simulink model "power_wind_dfig"  (R2016a)
settings: Solver=ode23tb  StartTime=0.0  StopTime=100  FixedStep=1/60  MaxStep=1/60  RelTol=1e-4  AbsTol=1e-3
InitFcn:
  | xInitial = init_power_wind_dfig;
undefined symbols (not defined in the file): b0, D1, D11, Delta, F, find_system, Fnom, gcbh, H, ILd_init, ILq_init, Imax_grid_conv, Init, j, Kd, Ki_dc_reg, Ki_grid_side_cur_reg, Ki_power_reg, Ki_Q, Ki_rotor_side_cur_reg, Ki_volt_reg, Kp, Kp_dc_reg, Kp_grid_side_cur_reg, Kp_power_reg, Kp_Q, Kp_rotor_side_cur_reg, Kp_volt_reg, L_RL, Llr, Lls, p, Pnom, power_A, power_B, power_D, R_RL, Rr, Rs, speed_A, speed_B, speed_C, speed_D, sps_rtmsupport, Vcontrol, Vnom, Wind_On, wo
libraries: powerlib_meascontrol x29, powerlib x27, simulink_extras x5, re_lib x2
(part 2 of 5)

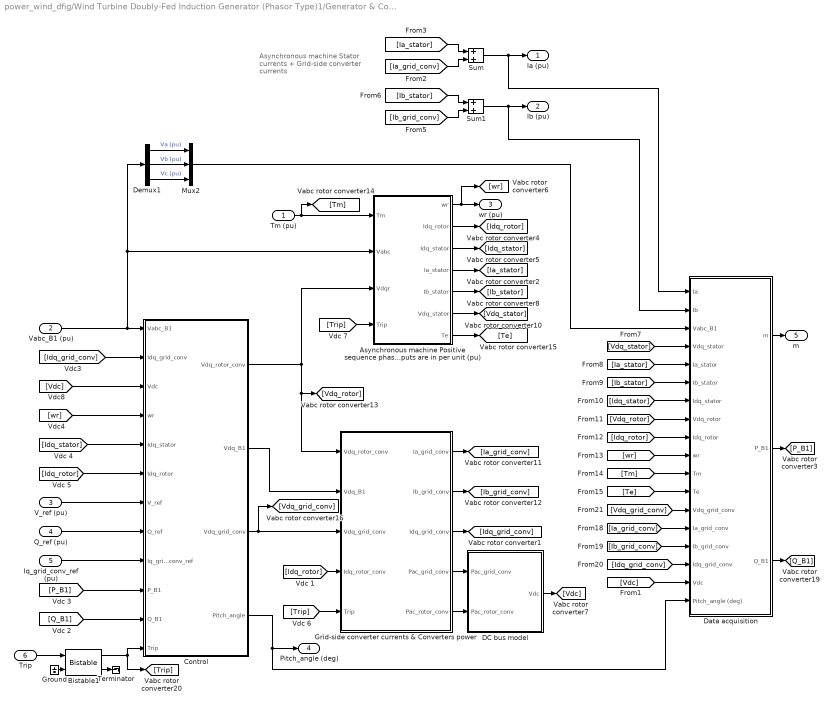
== system power_wind_dfig/Wind Turbine Doubly-Fed Induction Generator (Phasor Type)1/Generator & Converters ==
  note: Asynchronous machine
      | Stator currents
      | +
      | Grid-side converter
      | currents
  Tm (pu) : Inport
  Vabc_B1 (pu) : Inport  Port=2
  V_ref (pu) : Inport  Port=3
  Q_ref (pu) : Inport  Port=4
  Iq_grid_conv_ref (pu) : Inport  Port=5
  Trip : Inport  Port=6
  Asynchronous machine Positive sequence phasor model Inputs and outputs are in per unit (pu) : Subsystem  mask(Asynchronous Machine Model){nom=[ Pnom Vnom Fnom ], sta=[ Rs Lls], rot=[ Rr Llr], Lm=Lm, mec=[H F p], ini=init}
      mask prompts: nom "Nom. power,L-L volt. and freq. [ Pn(VA),Vn(Vrms),fn(Hz) ]:"; sta "Stator [ Rs,Lls (pu) ]:"; rot "Rotor [ Rr',Llr' (pu) ]:"; Lm "Magnetizing inductance Lm (pu):"; mec "Inertia constant,friction factor and pairs of poles [ H(s)  F(pu)  p() ]:"; ini "Initial conditions [s()  th(deg)  Is(pu)  ph_Is(deg)  Ir(pu)  ph_Ir(deg)]:"
      mask help: Implements a three-phase asynchronous machine (wound rotor) modelled in the dq stator reference frame. Stator and rotor windings are connected in wye to an internal neutral point.
      mask init:
      | %Initializes the Asynchronous Machine block before simulation.
      | 
      | % Base angular frequency
      | web=nom(3)*2*pi;
      | 
      | Rs=sta(1); Lls=sta(2);		% stator resistance and leakage inductance
      | Rr=rot(1); Llr=rot(2);		% rotor resistance and leakage inductance
      | Lm=Lm(1);			        % mutual inductance
      | H=mec(1); F=mec(2); p=mec(3);	% inertia, friction and pole pairs
      | s=ini(1);			% initial slip
      | wmo=1-s;			% initial speed
      | tho=ini(2)*pi/180;		% initial rotor angle
      | 
      | iso_mag=ini(3); iso_ph=ini(4)*pi/180; % init. stator current, phase A
      | iro_mag=ini(5); iro_ph=ini(6)*pi/180; % init. rotor current, phase A
      | 
      | % conversion of initial stator and rotor currents from polar to rectangular
      | % coordinates
      | [isdo,isqo]=pol2cart(iso_ph,iso_mag);
      | [irdo,irqo]=pol2cart(iro_ph,iro_mag);
      | 
      | % Initial fluxes (pu): inductances in pu, currents in pu
      | phisqo=((Lls+Lm)*isqo+Lm*irqo);
      | phisdo=((Lls+Lm)*isdo+Lm*irdo);
      | phirqo=((Llr+Lm)*irqo+Lm*isqo);
      | phirdo=((Llr+Lm)*irdo+Lm*isdo);
      | 
      | % Other inductances -------------------------------------------------------
      | 
      | Laq=1/(1/Lm+1/Lls+1/Llr);
      | Lad=Laq;
      mask Help: First 3 inputs: Stator terminals = phases a, b and c; 4th input: Simulink signal = Mechanical torque applied to the shaft (pu, >0 for motor mode, <0 for generator mode); First 3 outputs: Rotor terminals = phases a, b and c; 4th output: Simulink measurement output = vector (20x1) containing the following (all currents flowing into the machine): [1-3] : Rotor line currents ira, irb and irc; [4-5] : Rotor currents iqr and idr; [6-7] : Rotor fluxes phiqr and  phidr; [8-9] : Rotor voltages vqr and vdr; [10-12] : Stator line currents isa, isb, isc; [13-14] : Stator currents iqs and ids; [15-16] : Stator fluxes phiqs and  phids; [17-18] : Stator voltages vqs and vds; [19] : Rotor speed wm; [20 ]: Electromagnetic torque Te. Units of output measurement depend on checkbox in block's dialog box.
  Bistable1 : powerlib_meascontrol/Logic/Bistable  Qpriority=Set  ic=0  Ts=0
  Control : Subsystem
  DC bus model : Subsystem  mask(DC bus model){Pnom=Pnom, C=capacitor, Vdc_Init=Vdc_nom}
      mask prompts: Pnom "Nominal power (W):"; C "Capacitor (F):"; Vdc_Init "Initial voltage (V):"
  Data acquisition : Subsystem
  Demux1 : Demux  Outputs=3
  Grid-side converter currents & Converters power : Subsystem
  Ground : Ground
  Mux2 : Mux  Inputs=3
  Sum : Sum  SaturateOnIntegerOverflow=on
  Sum1 : Sum  SaturateOnIntegerOverflow=on
  Terminator : Terminator
  Ia (pu) : Outport
  Ib (pu) : Outport  Port=2
  wr (pu) : Outport  Port=3
  Pitch_angle (deg) : Outport  Port=4
  m : Outport  Port=5
  wires:
  Control/4(Pitch_angle) -> Pitch_angle (deg)/1, Data acquisition/18(Pitch_angle (deg))
  Bistable1/1 -> Control/12(Trip), [Trip]
  Ground/1 -> Bistable1/2
  Bistable1/2 -> Terminator/1
  Trip/1 -> Bistable1/1
  [Trip] -> Asynchronous machine Positive sequence phasor model Inputs and outputs are in per unit (pu)/4(Trip)
  [Trip] -> Grid-side converter currents & Converters power/5(Trip)
  V_ref (pu)/1 -> Control/7(V_ref)
  [Q_B1] -> Control/11(Q_B1)
  [P_B1] -> Control/10(P_B1)
  Data acquisition/2(P_B1) -> [P_B1]
  Iq_grid_conv_ref (pu)/1 -> Control/9(Iq_grid_conv_ref)
  Q_ref (pu)/1 -> Control/8(Q_ref)
  Data acquisition/3(Q_B1) -> [Q_B1]
  Demux1/3 -> Mux2/3  "Vc (pu)"
  Mux2/1 -> Data acquisition/3(Vabc_B1)
  Demux1/2 -> Mux2/2  "Vb (pu)"
  Demux1/1 -> Mux2/1  "Va (pu)"
  [Vdc] -> Data acquisition/17(Vdc)
  Data acquisition/1(m) -> m/1
  [Vdq_stator] -> Data acquisition/4(Vdq_stator)
  [Ia_stator] -> Data acquisition/5(Ia_stator)
  [Ib_stator] -> Data acquisition/6(Ib_stator)
  [Idq_stator] -> Data acquisition/7(Idq_stator)
  [Vdq_rotor] -> Data acquisition/8(Vdq_rotor)
  [Idq_rotor] -> Data acquisition/9(Idq_rotor)
  [wr] -> Data acquisition/10(wr)
  [Tm] -> Data acquisition/11(Tm)
  [Te] -> Data acquisition/12(Te)
  [Vdq_grid_conv] -> Data acquisition/13(Vdq_grid_conv)
  [Ia_grid_conv] -> Data acquisition/14(Ia_grid_conv)
  [Ib_grid_conv] -> Data acquisition/15(Ib_grid_conv)
  [Idq_grid_conv] -> Data acquisition/16(Idq_grid_conv)
  Asynchronous machine Positive sequence phasor model Inputs and outputs are in per unit (pu)/7(Te) -> [Te]
  [Ib_stator] -> Sum1/1
  [Ib_grid_conv] -> Sum1/2
  [Ia_stator] -> Sum/1
  [Ia_grid_conv] -> Sum/2
  Grid-side converter currents & Converters power/2(Ib_grid_conv) -> [Ib_grid_conv]
  Grid-side converter currents & Converters power/1(Ia_grid_conv) -> [Ia_grid_conv]
  Asynchronous machine Positive sequence phasor model Inputs and outputs are in per unit (pu)/6(Vdq_stator) -> [Vdq_stator]
  Asynchronous machine Positive sequence phasor model Inputs and outputs are in per unit (pu)/1(wr) -> [wr], wr (pu)/1
  Sum1/1 -> Data acquisition/2(Ib), Ib (pu)/1
  Sum/1 -> Data acquisition/1(Ia), Ia (pu)/1
  Vabc_B1 (pu)/1 -> Demux1/1, Asynchronous machine Positive sequence phasor model Inputs and outputs are in per unit (pu)/2(Vabc), Control/1(Vabc_B1)
  Grid-side converter currents & Converters power/5(Pac_rotor_conv) -> DC bus model/2(Pac_rotor_conv)
  Grid-side converter currents & Converters power/4(Pac_grid_conv) -> DC bus model/1(Pac_grid_conv)
  [Idq_rotor] -> Grid-side converter currents & Converters power/4(Idq_rotor_conv)
  Asynchronous machine Positive sequence phasor model Inputs and outputs are in per unit (pu)/4(Ia_stator) -> [Ia_stator]
  Asynchronous machine Positive sequence phasor model Inputs and outputs are in per unit (pu)/5(Ib_stator) -> [Ib_stator]
  Tm (pu)/1 -> [Tm], Asynchronous machine Positive sequence phasor model Inputs and outputs are in per unit (pu)/1(Tm)
  Asynchronous machine Positive sequence phasor model Inputs and outputs are in per unit (pu)/2(Idq_rotor) -> [Idq_rotor]
  Asynchronous machine Positive sequence phasor model Inputs and outputs are in per unit (pu)/3(Idq_stator) -> [Idq_stator]
  [Idq_grid_conv] -> Control/2(Idq_grid_conv)
  Grid-side converter currents & Converters power/3(Idq_grid_conv) -> [Idq_grid_conv]
  Control/2(Vdq_B1) -> Grid-side converter currents & Converters power/2(Vdq_B1)
  Control/1(Vdq_rotor_conv) -> [Vdq_rotor], Grid-side converter currents & Converters power/1(Vdq_rotor_conv), Asynchronous machine Positive sequence phasor model Inputs and outputs are in per unit (pu)/3("Vdqr ")
  Control/3(Vdq_grid_conv) -> [Vdq_grid_conv], Grid-side converter currents & Converters power/3(Vdq_grid_conv)
  [wr] -> Control/4(wr)
  [Vdc] -> Control/3(Vdc)
  [Idq_stator] -> Control/5(Idq_stator)
  [Idq_rotor] -> Control/6(Idq_rotor)
  DC bus model/1(Vdc) -> [Vdc]

== system power_wind_dfig/Wind Turbine Protection/Protection System ==
  Vabc (pu) : Inport  PortDimensions=3
  Iabc (pu) : Inport  Port=2  PortDimensions=3
  Vdc (V) : Inport  Port=3  PortDimensions=1
  Reset : Inport  Port=4  PortDimensions=1
  Speed (pu) : Inport  Port=5  PortDimensions=1
  AC Current Protection : Subsystem
  AC Voltage Protection : Subsystem
  Bistable1 : powerlib_meascontrol/Logic/Bistable  Qpriority=Set  ic=0  Ts=0
  Clock : Clock
  Constant : Constant  Value=Delay_Protection
  DC Voltage Protection : Subsystem
  Decoding : Subsystem
  Encoding : Subsystem
  Logical Operator : Logic  Operator=OR  Inputs=10  AllPortsSameDT=off
  Logical Operator1 : Logic  AllPortsSameDT=off
  Logical Operator2 : Logic  Operator=NOT  AllPortsSameDT=off
  Logical Operator3 : Logic  AllPortsSameDT=off
  Memory : Memory  InheritSampleTime=on
  Memory1 : Memory  InheritSampleTime=on
  Monostable1 : powerlib_meascontrol/Logic/Monostable  EdgeDetect=Rising  PulseDuration=1e-9  ic=0  Ts=0
  Relational Operator10 : RelationalOperator
  Sample & Hold : Subsystem  DialogController=POWERSYS.PowerSysDialog  mask(Sample & Hold){ic=0}
      mask prompts: ic "Initial condition:"
      mask help: The output follows input 1 (In) as long as input 2 (S) is TRUE (1) . The output is held when input 2 becomes FALSE (0). The output initial value is specified by the parameter "Initial condition".
      mask init:
      | power_initmask();
      mask Help: This block is part of a subset of blocks in the Extras library that does not have documentation associated with it, other than the block mask description.
      mask Display: disp('S/H')
  Sample & Hold1 : Subsystem  DialogController=POWERSYS.PowerSysDialog  mask(Sample & Hold){ic=0}
      mask prompts: ic "Initial condition:"
      mask help: The output follows input 1 (In) as long as input 2 (S) is TRUE (1) . The output is held when input 2 becomes FALSE (0). The output initial value is specified by the parameter "Initial condition".
      mask init:
      | power_initmask();
      mask Help: This block is part of a subset of blocks in the Extras library that does not have documentation associated with it, other than the block mask description.
      mask Display: disp('S/H')
  Terminator : Terminator
  Under/Over Speed Protection : Subsystem
  Trip : Outport
  TripTime : Outport  Port=2
  TripStatus : Outport  Port=3
  wires:
  Speed (pu)/1 -> Under/Over Speed Protection/1(Speed)
  Under/Over Speed Protection/2(MaxSpeed) -> Encoding/10(In10), Logical Operator/10
  Under/Over Speed Protection/1(MinSpeed) -> Encoding/9(In9), Logical Operator/9
  Relational Operator10/1 -> Logical Operator1/2
  Logical Operator/1 -> Logical Operator1/1
  Clock/1 -> Sample & Hold1/1(In), Relational Operator10/1
  Constant/1 -> Relational Operator10/2
  Monostable1/1 -> Sample & Hold1/2(S), Sample & Hold/2(S)
  Sample & Hold1/1("   ") -> TripTime/1
  AC Voltage Protection/4(MaxV0V1) -> Encoding/7(In7), Logical Operator/7
  AC Voltage Protection/3(MaxV2V1) -> Encoding/6(In6), Logical Operator/6
  AC Voltage Protection/2(MaxV1) -> Encoding/5(In5), Logical Operator/5
  AC Voltage Protection/1(MinV1) -> Encoding/4(In4), Logical Operator/4
  AC Current Protection/3(MaxI2I1) -> Encoding/3(In3), Logical Operator/3
  AC Current Protection/2(MaxI1) -> Encoding/2(In2), Logical Operator/2
  AC Current Protection/1(MaxIinst) -> Encoding/1(In1), Logical Operator/1
  Vabc (pu)/1 -> AC Voltage Protection/1(abc)
  Iabc (pu)/1 -> AC Current Protection/1(abc)
  Decoding/1(Out) -> TripStatus/1
  Sample & Hold/1("   ") -> Decoding/1(Code)
  Bistable1/2 -> Terminator/1
  Memory/1 -> Monostable1/1, Memory1/1
  Bistable1/1 -> Memory/1
  Encoding/1(Code) -> Sample & Hold/1(In)
  Logical Operator1/1 -> Bistable1/1, Logical Operator2/1
  Logical Operator3/1 -> Bistable1/2
  Reset/1 -> Logical Operator3/2
  Logical Operator2/1 -> Logical Operator3/1
  DC Voltage Protection/1(MaxVdc) -> Encoding/8(In8), Logical Operator/8
  Vdc (V)/1 -> DC Voltage Protection/1(Vdc)
  Memory1/1 -> Trip/1

== system power_wind_dfig/Measurements/Grid Data acquisition/Mean Value1 ==
  note: Mean value
  In : Inport
  Init : Inport  Port=2
  Gain : Gain  Gain=1/Period  SaturateOnIntegerOverflow=on  OutDataTypeStr=Inherit: Same as input  ParamDataTypeStr=Inherit: Same as input
  Step : Step  Time=Period+eps  SampleTime=0
  Sum : Sum  Inputs=+-  SaturateOnIntegerOverflow=on  InputSameDT=on  OutDataTypeStr=Inherit: Same as first input
  Switch : Switch  Threshold=0.5  SaturateOnIntegerOverflow=on
  Transport Delay : TransportDelay  DelayTime=Period
  integrator : Integrator
  Mean : Outport
  wires:
  Transport Delay/1 -> Sum/2
  integrator/1 -> Transport Delay/1, Sum/1
  In/1 -> integrator/1
  Sum/1 -> Gain/1
  Gain/1 -> Switch/1
  Switch/1 -> Mean/1
  Step/1 -> Switch/2
  Init/1 -> Switch/3

== system power_wind_dfig/Measurements/Grid Data acquisition/Mean Value2 ==
  note: Mean value
  In : Inport
  Init : Inport  Port=2
  Gain : Gain  Gain=1/Period  SaturateOnIntegerOverflow=on  OutDataTypeStr=Inherit: Same as input  ParamDataTypeStr=Inherit: Same as input
  Step : Step  Time=Period+eps  SampleTime=0
  Sum : Sum  Inputs=+-  SaturateOnIntegerOverflow=on  InputSameDT=on  OutDataTypeStr=Inherit: Same as first input
  Switch : Switch  Threshold=0.5  SaturateOnIntegerOverflow=on
  Transport Delay : TransportDelay  DelayTime=Period
  integrator : Integrator
  Mean : Outport
  wires:
  Init/1 -> Switch/3
  Step/1 -> Switch/2
  Switch/1 -> Mean/1
  Gain/1 -> Switch/1
  Sum/1 -> Gain/1
  In/1 -> integrator/1
  integrator/1 -> Sum/1, Transport Delay/1
  Transport Delay/1 -> Sum/2

== system power_wind_dfig/Measurements/Wind turbine Data acquisition/Mean Value1 ==
  note: Mean value
  In : Inport
  Init : Inport  Port=2
  Gain : Gain  Gain=1/Period  SaturateOnIntegerOverflow=on  OutDataTypeStr=Inherit: Same as input  ParamDataTypeStr=Inherit: Same as input
  Step : Step  Time=Period+eps  SampleTime=0
  Sum : Sum  Inputs=+-  SaturateOnIntegerOverflow=on  InputSameDT=on  OutDataTypeStr=Inherit: Same as first input
  Switch : Switch  Threshold=0.5  SaturateOnIntegerOverflow=on
  Transport Delay : TransportDelay  DelayTime=Period
  integrator : Integrator
  Mean : Outport
  wires:
  Transport Delay/1 -> Sum/2
  integrator/1 -> Transport Delay/1, Sum/1
  In/1 -> integrator/1
  Sum/1 -> Gain/1
  Gain/1 -> Switch/1
  Switch/1 -> Mean/1
  Step/1 -> Switch/2
  Init/1 -> Switch/3

== system power_wind_dfig/Measurements/Wind turbine Data acquisition/Mean Value2 ==
  note: Mean value
  In : Inport
  Init : Inport  Port=2
  Gain : Gain  Gain=1/Period  SaturateOnIntegerOverflow=on  OutDataTypeStr=Inherit: Same as input  ParamDataTypeStr=Inherit: Same as input
  Step : Step  Time=Period+eps  SampleTime=0
  Sum : Sum  Inputs=+-  SaturateOnIntegerOverflow=on  InputSameDT=on  OutDataTypeStr=Inherit: Same as first input
  Switch : Switch  Threshold=0.5  SaturateOnIntegerOverflow=on
  Transport Delay : TransportDelay  DelayTime=Period
  integrator : Integrator
  Mean : Outport
  wires:
  Init/1 -> Switch/3
  Step/1 -> Switch/2
  Switch/1 -> Mean/1
  Gain/1 -> Switch/1
  Sum/1 -> Gain/1
  In/1 -> integrator/1
  integrator/1 -> Sum/1, Transport Delay/1
  Transport Delay/1 -> Sum/2

== system power_wind_dfig/Measurements/Wind turbine Data acquisition/magnitude positive seq.  ==
  In1 : Inport
  Complex to Real-Imag : ComplexToRealImag
  Fourier1 : Subsystem  mask(Fourier analyser){f1=60, n=0}
      mask prompts: f1 "Fundamental frequency f1 (Hz):"; n "Harmonic n (0=DC; 1=fundamental; 2=2nd harm;  ...) :"
      mask help: The Fourier block performs a Fourier analysis of the input signal over a running window of one cycle of the fundamental frequency. First and second outputs return respectively the magnitude and phase (degrees) of the harmonic component specified.
      mask init:
      | k=2-(n==0);
      mask Help: helpview(psbhelp)
  Fourier2 : Subsystem  mask(Fourier analyser){f1=60, n=0}
      mask prompts: f1 "Fundamental frequency f1 (Hz):"; n "Harmonic n (0=DC; 1=fundamental; 2=2nd harm;  ...) :"
      mask help: The Fourier block performs a Fourier analysis of the input signal over a running window of one cycle of the fundamental frequency. First and second outputs return respectively the magnitude and phase (degrees) of the harmonic component specified.
      mask init:
      | k=2-(n==0);
      mask Help: helpview(psbhelp)
  Math Function : Math  Operator=hypot  SaturateOnIntegerOverflow=on
  Terminator : Terminator
  Terminator1 : Terminator
  Out1 : Outport
  wires:
  In1/1 -> Complex to Real-Imag/1
  Math Function/1 -> Out1/1
  Fourier2/1(magnitude) -> Math Function/2
  Fourier1/1(magnitude) -> Math Function/1
  Fourier2/2(angle) -> Terminator1/1
  Fourier1/2(angle) -> Terminator/1
  Complex to Real-Imag/2 -> Fourier2/1(signal)
  Complex to Real-Imag/1 -> Fourier1/1(signal)

== system power_wind_dfig/Measurements/Wind turbine Data acquisition/magnitude positivie seq ==
  In1 : Inport
  Complex to Real-Imag : ComplexToRealImag
  Fourier1 : Subsystem  mask(Fourier analyser){f1=60, n=0}
      mask prompts: f1 "Fundamental frequency f1 (Hz):"; n "Harmonic n (0=DC; 1=fundamental; 2=2nd harm;  ...) :"
      mask help: The Fourier block performs a Fourier analysis of the input signal over a running window of one cycle of the fundamental frequency. First and second outputs return respectively the magnitude and phase (degrees) of the harmonic component specified.
      mask init:
      | k=2-(n==0);
      mask Help: helpview(psbhelp)
  Fourier2 : Subsystem  mask(Fourier analyser){f1=60, n=0}
      mask prompts: f1 "Fundamental frequency f1 (Hz):"; n "Harmonic n (0=DC; 1=fundamental; 2=2nd harm;  ...) :"
      mask help: The Fourier block performs a Fourier analysis of the input signal over a running window of one cycle of the fundamental frequency. First and second outputs return respectively the magnitude and phase (degrees) of the harmonic component specified.
      mask init:
      | k=2-(n==0);
      mask Help: helpview(psbhelp)
  Math Function : Math  Operator=hypot  SaturateOnIntegerOverflow=on
  Terminator : Terminator
  Terminator1 : Terminator
  Out1 : Outport
  wires:
  Complex to Real-Imag/1 -> Fourier1/1(signal)
  Complex to Real-Imag/2 -> Fourier2/1(signal)
  Fourier1/2(angle) -> Terminator/1
  Fourier2/2(angle) -> Terminator1/1
  Fourier1/1(magnitude) -> Math Function/1
  Fourier2/1(magnitude) -> Math Function/2
  Math Function/1 -> Out1/1
  In1/1 -> Complex to Real-Imag/1

== system power_wind_dfig/Plant 2 MVA/Plant & Motor Protection/AC Current Protection ==
  abc : Inport  PortDimensions=3
  Complex to Magnitude-Angle1 : ComplexToMagnitudeAngle  Output=Magnitude
  Current Measurement : Subsystem
  MinMax : MinMax  Function=max  ZeroCross=off  SaturateOnIntegerOverflow=on  InputSameDT=on
  Mux : Mux  Inputs=3
  On Delay : powerlib_meascontrol/Logic/On Delay  DelayType=On delay  delay=Delay_I1  ic=0  Ts=0
  On Delay1 : powerlib_meascontrol/Logic/On Delay  DelayType=On delay  delay=Delay_I2_I1  ic=0  Ts=0
  Relational Operator10 : RelationalOperator  Operator=>
  Relational Operator6 : RelationalOperator  Operator=>
  Relational Operator8 : RelationalOperator  Operator=>
  Selector : Selector  InputPortWidth=3  IndexOptions=Index vector (dialog)  Indices=1  OutputSizes=1
  Selector1 : Selector  InputPortWidth=3  IndexOptions=Index vector (dialog)  Indices=2  OutputSizes=1
  Selector2 : Selector  InputPortWidth=3  IndexOptions=Index vector (dialog)  Indices=3  OutputSizes=1
  V0/V1 max3 : Constant  Value=Max_I1
  V1 max : Constant  Value=Max_I2_I1
  V1 max2 : Constant  Value=Max_Iinst
  MaxIinst : Outport
  MaxI1 : Outport  Port=2
  MaxI2I1 : Outport  Port=3
  wires:
  MinMax/1 -> Relational Operator10/1
  Complex to Magnitude-Angle1/1 -> MinMax/1
  Mux/1 -> Complex to Magnitude-Angle1/1
  Selector1/1 -> Mux/2
  Selector2/1 -> Mux/3
  Selector/1 -> Mux/1
  V1 max2/1 -> Relational Operator10/2
  Relational Operator10/1 -> MaxIinst/1
  On Delay1/1 -> MaxI2I1/1
  On Delay/1 -> MaxI1/1
  Relational Operator8/1 -> On Delay1/1
  Relational Operator6/1 -> On Delay/1
  Current Measurement/2(I2/I1) -> Relational Operator8/1
  V1 max/1 -> Relational Operator8/2
  V0/V1 max3/1 -> Relational Operator6/2
  Current Measurement/1(I1) -> Relational Operator6/1
  abc/1 -> Selector2/1, Selector1/1, Selector/1, Current Measurement/1(abc)

== system power_wind_dfig/Plant 2 MVA/Plant & Motor Protection/AC Voltage Protection ==
  abc : Inport  PortDimensions=3
  On Delay : powerlib_meascontrol/Logic/On Delay  DelayType=On delay  delay=Delay_V1  ic=0  Ts=0
  On Delay1 : powerlib_meascontrol/Logic/On Delay  DelayType=On delay  delay=Delay_V2_V1  ic=0  Ts=0
  On Delay2 : powerlib_meascontrol/Logic/On Delay  DelayType=On delay  delay=Delay_V1  ic=0  Ts=0
  On Delay3 : powerlib_meascontrol/Logic/On Delay  DelayType=On delay  delay=Delay_V2_V1  ic=0  Ts=0
  Relational Operator6 : RelationalOperator  Operator=>
  Relational Operator7 : RelationalOperator  Operator=<
  Relational Operator8 : RelationalOperator  Operator=>
  Relational Operator9 : RelationalOperator  Operator=>
  V0/V1 max3 : Constant  Value=Max_V1
  V0/V1 max4 : Constant  Value=Min_V1
  V1 max : Constant  Value=Max_V2_V1
  V1 max1 : Constant  Value=Max_V0_V1
  Voltage Measurement : Subsystem
  MinV1 : Outport
  MaxV1 : Outport  Port=2
  MaxV2V1 : Outport  Port=3
  MaxV0V1 : Outport  Port=4
  wires:
  abc/1 -> Voltage Measurement/1(abc)
  Voltage Measurement/1(V1) -> Relational Operator6/1, Relational Operator7/1
  V0/V1 max3/1 -> Relational Operator6/2
  V0/V1 max4/1 -> Relational Operator7/2
  V1 max/1 -> Relational Operator8/2
  Voltage Measurement/2(V2/V1) -> Relational Operator8/1
  V1 max1/1 -> Relational Operator9/2
  Voltage Measurement/3(V0/V1) -> Relational Operator9/1
  Relational Operator6/1 -> On Delay2/1
  Relational Operator7/1 -> On Delay/1
  Relational Operator8/1 -> On Delay1/1
  Relational Operator9/1 -> On Delay3/1
  On Delay2/1 -> MaxV1/1
  On Delay/1 -> MinV1/1
  On Delay1/1 -> MaxV2V1/1
  On Delay3/1 -> MaxV0V1/1

== system power_wind_dfig/Plant 2 MVA/Plant & Motor Protection/DC Voltage Protection ==
  Vdc : Inport
  On Delay : powerlib_meascontrol/Logic/On Delay  DelayType=On delay  delay=Delay_Vdc  ic=0  Ts=0
  Relational Operator1 : RelationalOperator  Operator=>
  V1 max3 : Constant  Value=Max_Vdc
  MaxVdc : Outport
  wires:
  On Delay/1 -> MaxVdc/1
  Relational Operator1/1 -> On Delay/1
  V1 max3/1 -> Relational Operator1/2
  Vdc/1 -> Relational Operator1/1

== system power_wind_dfig/Plant 2 MVA/Plant & Motor Protection/Decoding ==
  Code : Inport
  Constant : Constant  Value=pow2(0:-1:-9)
  Constant6 : Constant  Value=2
  Math Function : Math  Operator=rem  SaturateOnIntegerOverflow=on
  Product : Product  SaturateOnIntegerOverflow=on  InputSameDT=on  OutDataTypeStr=Inherit: Same as first input
  Rounding Function : Rounding
  Out : Outport
  wires:
  Math Function/1 -> Out/1
  Rounding Function/1 -> Math Function/1
  Constant6/1 -> Math Function/2
  Product/1 -> Rounding Function/1
  Code/1 -> Product/1
  Constant/1 -> Product/2

== system power_wind_dfig/Plant 2 MVA/Plant & Motor Protection/Encoding ==
  In1 : Inport
  In2 : Inport  Port=2
  In3 : Inport  Port=3
  In4 : Inport  Port=4
  In5 : Inport  Port=5
  In6 : Inport  Port=6
  In7 : Inport  Port=7
  In8 : Inport  Port=8
  In9 : Inport  Port=9
  In10 : Inport  Port=10
  Constant12 : Constant  Value=pow2(0:1:9)
  Data Type Conversion : DataTypeConversion  SaturateOnIntegerOverflow=on  RndMeth=Zero
  Mux : Mux  Inputs=10
  Product : Product  SaturateOnIntegerOverflow=on  InputSameDT=on  OutDataTypeStr=Inherit: Same as first input
  Sum : Sum  Inputs=1  SaturateOnIntegerOverflow=on  InputSameDT=on  OutDataTypeStr=Inherit: Same as first input
  Code : Outport
  wires:
  Sum/1 -> Code/1
  Constant12/1 -> Product/2
  Product/1 -> Sum/1
  In1/1 -> Mux/1
  In10/1 -> Mux/10
  In9/1 -> Mux/9
  In8/1 -> Mux/8
  In7/1 -> Mux/7
  In6/1 -> Mux/6
  In5/1 -> Mux/5
  In4/1 -> Mux/4
  In3/1 -> Mux/3
  In2/1 -> Mux/2
  Mux/1 -> Data Type Conversion/1
  Data Type Conversion/1 -> Product/1

== system power_wind_dfig/Plant 2 MVA/Plant & Motor Protection/Sample & Hold ==
  note: Silvano Casoria
      | Power System Simulation Laboratory
      | IREQ, Hydro-Quebc
  note: Sample and Hold
  In : Inport
  S : Inport  Port=2
  IC=ic : Memory  X0=ic  InheritSampleTime=on
  Switch : Switch  Threshold=0.5  SaturateOnIntegerOverflow=on  InputSameDT=on
  "   " : Outport  InitialOutput=0
  wires:
  S/1 -> Switch/2
  In/1 -> Switch/1
  IC=ic/1 -> Switch/3
  Switch/1 -> IC=ic/1, "   "/1

== system power_wind_dfig/Plant 2 MVA/Plant & Motor Protection/Sample & Hold1 ==
  note: Silvano Casoria
      | Power System Simulation Laboratory
      | IREQ, Hydro-Quebc
  note: Sample and Hold
  In : Inport
  S : Inport  Port=2
  IC=ic : Memory  X0=ic  InheritSampleTime=on
  Switch : Switch  Threshold=0.5  SaturateOnIntegerOverflow=on  InputSameDT=on
  "   " : Outport  InitialOutput=0
  wires:
  S/1 -> Switch/2
  In/1 -> Switch/1
  IC=ic/1 -> Switch/3
  Switch/1 -> IC=ic/1, "   "/1

== system power_wind_dfig/Plant 2 MVA/Plant & Motor Protection/Under//Over Speed Protection ==
  Speed : Inport  PortDimensions=1
  On Delay : powerlib_meascontrol/Logic/On Delay  DelayType=On delay  delay=Delay_Speed  ic=0  Ts=0
  On Delay1 : powerlib_meascontrol/Logic/On Delay  DelayType=On delay  delay=Delay_Speed  ic=0  Ts=0
  Relational Operator1 : RelationalOperator  Operator=>
  Relational Operator3 : RelationalOperator  Operator=<
  V1 max1 : Constant  Value=Min_Speed
  V1 max3 : Constant  Value=Max_Speed
  MinSpeed : Outport
  MaxSpeed : Outport  Port=2
  wires:
  Speed/1 -> Relational Operator1/1, Relational Operator3/1
  V1 max3/1 -> Relational Operator1/2
  V1 max1/1 -> Relational Operator3/2
  Relational Operator1/1 -> On Delay1/1
  Relational Operator3/1 -> On Delay/1
  On Delay/1 -> MinSpeed/1
  On Delay1/1 -> MaxSpeed/1

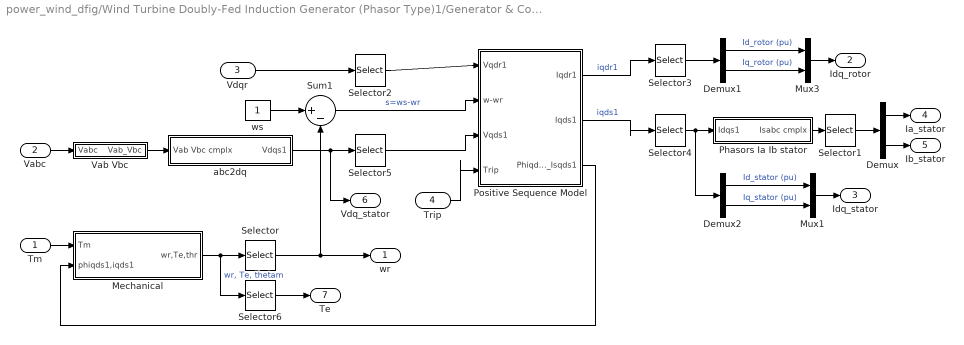
== system power_wind_dfig/Wind Turbine Doubly-Fed Induction Generator (Phasor Type)1/Generator & Converters/Asynchronous machine Positive sequence phasor model Inputs and outputs are in per unit (pu) ==
  Tm : Inport
  Vabc : Inport  Port=2
  "Vdqr " : Inport  Port=3
  Trip : Inport  Port=4
  Demux : Demux  Outputs=2
  Demux1 : Demux  Outputs=2
  Demux2 : Demux  Outputs=2
  Mechanical : Subsystem
  Mux1 : Mux  Inputs=2
  Mux3 : Mux  Inputs=2
  Phasors Ia Ib stator : Subsystem
  Positive Sequence Model : Subsystem
  Selector : Selector  InputPortWidth=3  IndexOptions=Index vector (dialog)  Indices=1  OutputSizes=1
  Selector1 : Selector  InputPortWidth=3  IndexOptions=Index vector (dialog)  Indices=[1 2]  OutputSizes=1
  Selector{2..5} (4 alike) : Selector  InputPortWidth=2  IndexOptions=Index vector (dialog)  Indices=[2 1]  OutputSizes=1
  Selector6 : Selector  InputPortWidth=3  IndexOptions=Index vector (dialog)  Indices=2  OutputSizes=1
  Sum1 : Sum  Inputs=|+-  SaturateOnIntegerOverflow=on  InputSameDT=on  OutDataTypeStr=Inherit: Same as first input
  Vab Vbc : Subsystem
  abc2dq : Subsystem
  ws : Constant
  wr : Outport
  Idq_rotor : Outport  Port=2
  Idq_stator : Outport  Port=3
  Ia_stator : Outport  Port=4
  Ib_stator : Outport  Port=5
  Vdq_stator : Outport  Port=6
  Te : Outport  Port=7
  wires:
  Trip/1 -> Positive Sequence Model/4(Trip)
  Positive Sequence Model/3(Phiqds1_Isqds1) -> Mechanical/2(phiqds1,iqds1)
  Positive Sequence Model/2(Iqds1) -> Selector4/1  "iqds1"
  Positive Sequence Model/1(Iqdr1) -> Selector3/1  "iqdr1"
  Mux1/1 -> Idq_stator/1
  Demux2/2 -> Mux1/2  "Iq_stator (pu)"
  Demux2/1 -> Mux1/1  "Id_stator (pu)"
  Mux3/1 -> Idq_rotor/1
  Demux1/2 -> Mux3/2  "Iq_rotor (pu)"
  Demux1/1 -> Mux3/1  "Id_rotor (pu)"
  Selector3/1 -> Demux1/1
  Selector6/1 -> Te/1
  Selector1/1 -> Demux/1
  Demux/2 -> Ib_stator/1
  Demux/1 -> Ia_stator/1
  Tm/1 -> Mechanical/1(Tm)
  Phasors Ia Ib stator/1(Isabc cmplx) -> Selector1/1
  Vabc/1 -> Vab Vbc/1(Vabc)
  Vab Vbc/1(Vab_Vbc) -> abc2dq/1(Vab Vbc cmplx)
  abc2dq/1(Vdqs1) -> Vdq_stator/1, Selector5/1
  "Vdqr "/1 -> Selector2/1
  Mechanical/1(wr,Te,thr) -> Selector6/1, Selector/1  "wr, Te, thetam"
  ws/1 -> Sum1/1
  Selector/1 -> Sum1/2, wr/1
  Sum1/1 -> Positive Sequence Model/2(w-wr)  "s=ws-wr"
  Selector2/1 -> Positive Sequence Model/1(Vqdr1)
  Selector5/1 -> Positive Sequence Model/3(Vqds1)
  Selector4/1 -> Demux2/1, Phasors Ia Ib stator/1(Idqs1)

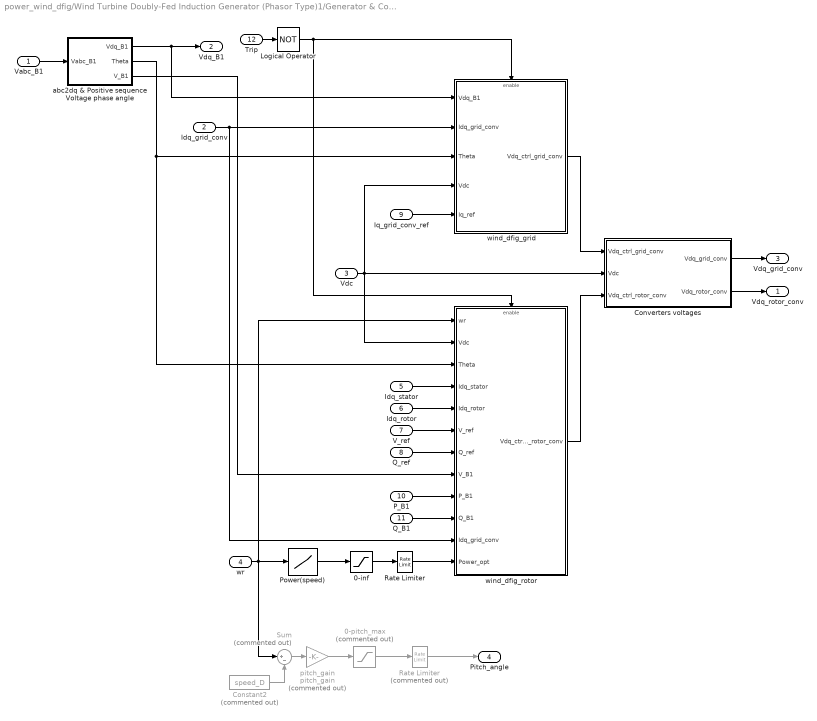
== system power_wind_dfig/Wind Turbine Doubly-Fed Induction Generator (Phasor Type)1/Generator & Converters/Control ==
  Vabc_B1 : Inport
  Idq_grid_conv : Inport  Port=2
  Vdc : Inport  Port=3
  wr : Inport  Port=4
  Idq_stator : Inport  Port=5
  Idq_rotor : Inport  Port=6
  V_ref : Inport  Port=7  SampleTime=0
  Q_ref : Inport  Port=8  SampleTime=0
  Iq_grid_conv_ref : Inport  Port=9  SampleTime=0
  P_B1 : Inport  Port=10
  Q_B1 : Inport  Port=11
  Trip : Inport  Port=12
  0-inf : Saturate  UpperLimit=inf  LowerLimit=0
  0-pitch_max : Saturate  Commented=on  UpperLimit=pitch_max  LowerLimit=0
  Constant2 : Constant  Commented=on  Value=speed_D
  Converters voltages : Subsystem
  Logical Operator : Logic  Operator=NOT  AllPortsSameDT=off  OutDataTypeStr=float('double')  SampleTime=0
  Power(speed) : Lookup  InputValues=speed_power(:,1)  Table=speed_power(:,2)  SaturateOnIntegerOverflow=on
  "Rate Limiter " : RateLimiter  RisingSlewLimit=power_slew_rate  FallingSlewLimit=-power_slew_rate
  "Rate Limiter   " : RateLimiter  Commented=on  RisingSlewLimit=pitch_rate  FallingSlewLimit=-pitch_rate
  Sum : Sum  Commented=on  Inputs=|+-  SaturateOnIntegerOverflow=on
  abc2dq & Positive sequence Voltage phase angle : Subsystem
  pitch_gain : Gain  Commented=on  Gain=pitch_gain  SaturateOnIntegerOverflow=on  OutDataTypeStr=Inherit: Same as input  ParamDataTypeStr=Inherit: Same as input
  wind_dfig_grid : Subsystem
  wind_dfig_rotor : Subsystem
  Vdq_rotor_conv : Outport
  Vdq_B1 : Outport  Port=2
  Vdq_grid_conv : Outport  Port=3
  Pitch_angle : Outport  Port=4
  wires:
  Logical Operator/1 -> wind_dfig_rotor/Enable, wind_dfig_grid/Enable
  wind_dfig_rotor/1(Vdq_ctrl_rotor_conv) -> Converters voltages/3(Vdq_ctrl_rotor_conv)
  "Rate Limiter   "/1 -> Pitch_angle/1
  pitch_gain/1 -> 0-pitch_max/1
  Sum/1 -> pitch_gain/1
  Constant2/1 -> Sum/2
  0-pitch_max/1 -> "Rate Limiter   "/1
  "Rate Limiter "/1 -> wind_dfig_rotor/12(Power_opt)
  Power(speed)/1 -> 0-inf/1
  0-inf/1 -> "Rate Limiter "/1
  wind_dfig_grid/1(Vdq_ctrl_grid_conv) -> Converters voltages/1(Vdq_ctrl_grid_conv)
  Trip/1 -> Logical Operator/1
  Q_B1/1 -> wind_dfig_rotor/10(Q_B1)
  P_B1/1 -> wind_dfig_rotor/9(P_B1)
  wr/1 -> wind_dfig_rotor/1(wr), Sum/1, Power(speed)/1
  abc2dq & Positive sequence Voltage phase angle/3(V_B1) -> wind_dfig_rotor/8(V_B1)
  Q_ref/1 -> wind_dfig_rotor/7(Q_ref)
  V_ref/1 -> wind_dfig_rotor/6(V_ref)
  Idq_rotor/1 -> wind_dfig_rotor/5(Idq_rotor)
  Idq_stator/1 -> wind_dfig_rotor/4(Idq_stator)
  Iq_grid_conv_ref/1 -> wind_dfig_grid/5(Iq_ref)
  Vabc_B1/1 -> abc2dq & Positive sequence Voltage phase angle/1(Vabc_B1)
  Idq_grid_conv/1 -> wind_dfig_rotor/11(Idq_grid_conv), wind_dfig_grid/2(Idq_grid_conv)
  Converters voltages/1(Vdq_grid_conv) -> Vdq_grid_conv/1
  Converters voltages/2(Vdq_rotor_conv) -> Vdq_rotor_conv/1
  abc2dq & Positive sequence Voltage phase angle/1(Vdq_B1) -> wind_dfig_grid/1(Vdq_B1), Vdq_B1/1
  abc2dq & Positive sequence Voltage phase angle/2(Theta) -> wind_dfig_rotor/3(Theta), wind_dfig_grid/3(Theta)
  Vdc/1 -> wind_dfig_rotor/2(Vdc), wind_dfig_grid/4(Vdc), Converters voltages/2(Vdc)

== system power_wind_dfig/Wind Turbine Doubly-Fed Induction Generator (Phasor Type)1/Generator & Converters/DC bus model ==
  note: Pdc = Pac_grid_conv - Pac_rotor_conv
  Pac_grid_conv : Inport
  Pac_rotor_conv : Inport  Port=2
  Integrator : Integrator  InitialCondition=Vdc_Init  LowerSaturationLimit=1e-6  ZeroCross=off
  Product2 : Product  Inputs=*/  SaturateOnIntegerOverflow=on  InputSameDT=on  OutDataTypeStr=Inherit: Same as first input
  Sum2 : Sum  Inputs=|+-  SaturateOnIntegerOverflow=on  InputSameDT=on  OutDataTypeStr=Inherit: Same as first input
  deg->rad1 : Gain  Gain=1/C  SaturateOnIntegerOverflow=on  OutDataTypeStr=Inherit: Same as input  ParamDataTypeStr=Inherit: Same as input
  pu->W : Gain  Gain=Pnom  SaturateOnIntegerOverflow=on  OutDataTypeStr=Inherit: Same as input  ParamDataTypeStr=Inherit: Same as input
  Vdc : Outport
  wires:
  Sum2/1 -> pu->W/1
  Pac_rotor_conv/1 -> Sum2/2
  Product2/1 -> deg->rad1/1  "Idc"
  Integrator/1 -> Product2/2, Vdc/1  "Vdc"
  deg->rad1/1 -> Integrator/1
  Pac_grid_conv/1 -> Sum2/1
  pu->W/1 -> Product2/1

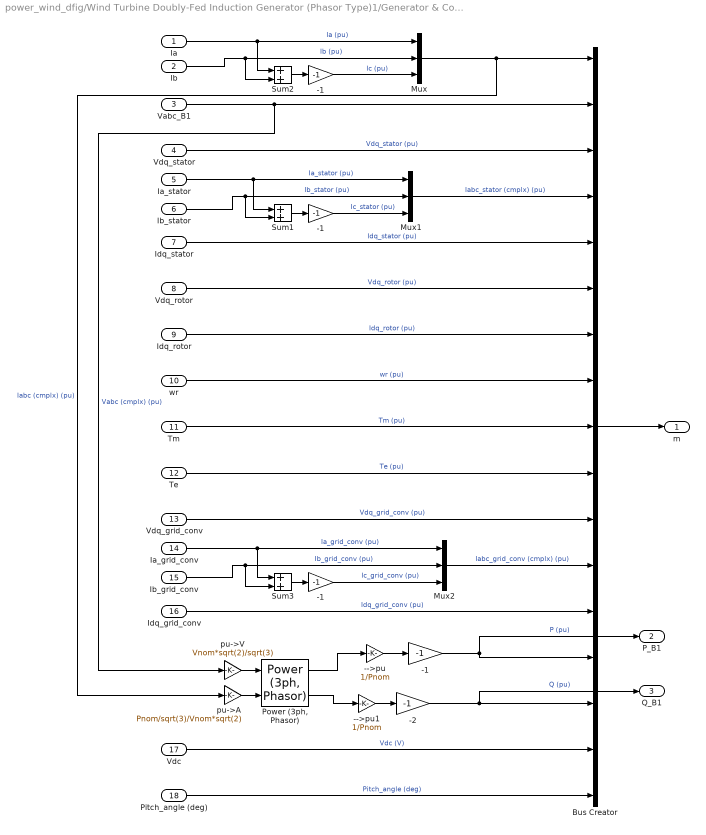
== system power_wind_dfig/Wind Turbine Doubly-Fed Induction Generator (Phasor Type)1/Generator & Converters/Data acquisition ==
  Ia : Inport
  Ib : Inport  Port=2
  Vabc_B1 : Inport  Port=3
  Vdq_stator : Inport  Port=4
  Ia_stator : Inport  Port=5
  Ib_stator : Inport  Port=6
  Idq_stator : Inport  Port=7
  Vdq_rotor : Inport  Port=8
  Idq_rotor : Inport  Port=9
  wr : Inport  Port=10
  Tm : Inport  Port=11
  Te : Inport  Port=12
  Vdq_grid_conv : Inport  Port=13
  Ia_grid_conv : Inport  Port=14
  Ib_grid_conv : Inport  Port=15
  Idq_grid_conv : Inport  Port=16
  Vdc : Inport  Port=17
  Pitch_angle (deg) : Inport  Port=18
  " -1" : Gain  Gain=-1  SaturateOnIntegerOverflow=on  OutDataTypeStr=Inherit: Same as input  ParamDataTypeStr=Inherit: Same as input
  -->pu : Gain  Gain=1/Pnom  SaturateOnIntegerOverflow=on  OutDataTypeStr=Inherit: Same as input  ParamDataTypeStr=Inherit: Same as input
  -->pu1 : Gain  Gain=1/Pnom  SaturateOnIntegerOverflow=on  OutDataTypeStr=Inherit: Same as input  ParamDataTypeStr=Inherit: Same as input
  -1 : Gain  Gain=-1  SaturateOnIntegerOverflow=on  OutDataTypeStr=Inherit: Same as input  ParamDataTypeStr=Inherit: Same as input
  "-1 " : Gain  Gain=-1  SaturateOnIntegerOverflow=on  OutDataTypeStr=Inherit: Same as input  ParamDataTypeStr=Inherit: Same as input
  "-1  " : Gain  Gain=-1  SaturateOnIntegerOverflow=on  OutDataTypeStr=Inherit: Same as input  ParamDataTypeStr=Inherit: Same as input
  -2 : Gain  Gain=-1  SaturateOnIntegerOverflow=on  OutDataTypeStr=Inherit: Same as input  ParamDataTypeStr=Inherit: Same as input
  Bus Creator : BusCreator  Inputs=17
  Mux : Mux  Inputs=3
  Mux1 : Mux  Inputs=3
  Mux2 : Mux  Inputs=3
  "Power (3ph, Phasor)" : powerlib_meascontrol/Measurements/Power (3ph, Phasor)
  Sum1 : Sum  SaturateOnIntegerOverflow=on
  Sum2 : Sum  SaturateOnIntegerOverflow=on
  Sum3 : Sum  SaturateOnIntegerOverflow=on
  pu->A : Gain  Gain=Pnom/sqrt(3)/Vnom*sqrt(2)  SaturateOnIntegerOverflow=on  OutDataTypeStr=Inherit: Same as input  ParamDataTypeStr=Inherit: Same as input
  pu->V : Gain  Gain=Vnom*sqrt(2)/sqrt(3)  SaturateOnIntegerOverflow=on  OutDataTypeStr=Inherit: Same as input  ParamDataTypeStr=Inherit: Same as input
  m : Outport
  P_B1 : Outport  Port=2
  Q_B1 : Outport  Port=3
  wires:
  "Power (3ph, Phasor)"/2 -> -->pu1/1
  "Power (3ph, Phasor)"/1 -> -->pu/1
  -->pu1/1 -> -2/1
  Bus Creator/1 -> m/1
  Pitch_angle (deg)/1 -> Bus Creator/17  "Pitch_angle (deg)"
  -1/1 -> P_B1/1, Bus Creator/14  "P (pu)"
  -2/1 -> Bus Creator/15, Q_B1/1  "Q (pu)"
  Vdc/1 -> Bus Creator/16  "Vdc (V)"
  Idq_grid_conv/1 -> Bus Creator/13  "Idq_grid_conv (pu)"
  Mux2/1 -> Bus Creator/12  "Iabc_grid_conv (cmplx) (pu)"
  Vdq_grid_conv/1 -> Bus Creator/11  "Vdq_grid_conv (pu)"
  Te/1 -> Bus Creator/10  "Te (pu)"
  Tm/1 -> Bus Creator/9  "Tm (pu)"
  wr/1 -> Bus Creator/8  "wr (pu)"
  Idq_rotor/1 -> Bus Creator/7  "Idq_rotor (pu)"
  Vdq_rotor/1 -> Bus Creator/6  "Vdq_rotor (pu)"
  Idq_stator/1 -> Bus Creator/5  "Idq_stator (pu)"
  Vdq_stator/1 -> Bus Creator/3  "Vdq_stator (pu)"
  Vabc_B1/1 -> Bus Creator/2, pu->V/1  "Vabc (cmplx) (pu)"
  Mux/1 -> Bus Creator/1, pu->A/1  "Iabc (cmplx) (pu)"
  Mux1/1 -> Bus Creator/4  "Iabc_stator (cmplx) (pu)"
  Ia_grid_conv/1 -> Mux2/1, Sum3/1  "Ia_grid_conv (pu)"
  Ib_grid_conv/1 -> Mux2/2, Sum3/2  "Ib_grid_conv (pu)"
  " -1"/1 -> Mux2/3  "Ic_grid_conv (pu)"
  Sum3/1 -> " -1"/1
  pu->V/1 -> "Power (3ph, Phasor)"/1
  Ia_stator/1 -> Sum1/1, Mux1/1  "Ia_stator (pu)"
  Ib_stator/1 -> Sum1/2, Mux1/2  "Ib_stator (pu)"
  "-1  "/1 -> Mux1/3  "Ic_stator (pu)"
  Sum1/1 -> "-1  "/1
  Ia/1 -> Mux/1, Sum2/1  "Ia (pu)"
  Ib/1 -> Mux/2, Sum2/2  "Ib (pu)"
  "-1 "/1 -> Mux/3  "Ic (pu)"
  Sum2/1 -> "-1 "/1
  -->pu/1 -> -1/1
  pu->A/1 -> "Power (3ph, Phasor)"/2

== system power_wind_dfig/Wind Turbine Doubly-Fed Induction Generator (Phasor Type)1/Generator & Converters/Grid-side converter currents & Converters power ==
  Vdq_rotor_conv : Inport
  Vdq_B1 : Inport  Port=2
  Vdq_grid_conv : Inport  Port=3
  Idq_rotor_conv : Inport  Port=4
  Trip : Inport  Port=5
  Demux : Demux  Outputs=2
  Demux1 : Demux  Outputs=2
  Mux2 : Mux  Inputs=2
  Product1 : Product  Inputs=**  SaturateOnIntegerOverflow=on  InputSameDT=on  OutDataTypeStr=Inherit: Same as first input
  Product3 : Product  Inputs=**  SaturateOnIntegerOverflow=on  InputSameDT=on  OutDataTypeStr=Inherit: Same as first input
  Sum1 : Sum  Inputs=1  SaturateOnIntegerOverflow=on  InputSameDT=on  OutDataTypeStr=Inherit: Same as first input
  Sum3 : Sum  Inputs=1  SaturateOnIntegerOverflow=on  InputSameDT=on  OutDataTypeStr=Inherit: Same as first input
  d-q axis model of a 3-phase series R-L branch : Subsystem  mask(d-q axis model of a 3-phase series R-L branch){R=R_RL, L=L_RL, Fnom=Fnom, Idq0=[ILd_init ILq_init]}
      mask prompts: R "R (pu)"; L "L (pu)"; Fnom "Nominal frequency (Hz)"; Idq0 "Initial currents [Id Iq] (pu)"
      mask help:
      | This block implements a d-q axis model of a 3-phase R-L branch.
      | Inputs:
      | d-q axis voltages (V1 and V2) at each terminal of the R-L branch in pu.
      | Outputs:
      | d-q axis currents flowing (from V1 to V2) in the R-L branch in pu.
      mask init:
      | w=2*pi*Fnom;
  dq2ab : Subsystem
  Ia_grid_conv : Outport
  Ib_grid_conv : Outport  Port=2
  Idq_grid_conv : Outport  Port=3
  Pac_grid_conv : Outport  Port=4
  Pac_rotor_conv : Outport  Port=5
  wires:
  Trip/1 -> d-q axis model of a 3-phase series R-L branch/3(Trip)
  Mux2/1 -> Idq_grid_conv/1
  Demux1/2 -> Mux2/2  "Iq_grid_conv (pu)"
  Demux1/1 -> Mux2/1  "Id_grid_conv (pu)"
  Vdq_B1/1 -> d-q axis model of a 3-phase series R-L branch/1(Vdq1)
  Vdq_grid_conv/1 -> Product3/2, d-q axis model of a 3-phase series R-L branch/2(Vdq2)
  Product3/1 -> Sum3/1
  Sum3/1 -> Pac_grid_conv/1
  Product1/1 -> Sum1/1
  Sum1/1 -> Pac_rotor_conv/1
  Vdq_rotor_conv/1 -> Product1/1
  Idq_rotor_conv/1 -> Product1/2
  d-q axis model of a 3-phase series R-L branch/1(Idq) -> Product3/1, Demux1/1, dq2ab/1(Idq_seq1)
  dq2ab/1(Ia_Ib complx) -> Demux/1
  Demux/1 -> Ia_grid_conv/1
  Demux/2 -> Ib_grid_conv/1

== system power_wind_dfig/Wind Turbine Protection/Protection System/AC Current Protection ==
  abc : Inport  PortDimensions=3
  Complex to Magnitude-Angle1 : ComplexToMagnitudeAngle  Output=Magnitude
  Current Measurement : Subsystem
  MinMax : MinMax  Function=max  ZeroCross=off  SaturateOnIntegerOverflow=on  InputSameDT=on
  Mux : Mux  Inputs=3
  On Delay : powerlib_meascontrol/Logic/On Delay  DelayType=On delay  delay=Delay_I1  ic=0  Ts=0
  On Delay1 : powerlib_meascontrol/Logic/On Delay  DelayType=On delay  delay=Delay_I2_I1  ic=0  Ts=0
  Relational Operator10 : RelationalOperator  Operator=>
  Relational Operator6 : RelationalOperator  Operator=>
  Relational Operator8 : RelationalOperator  Operator=>
  Selector : Selector  InputPortWidth=3  IndexOptions=Index vector (dialog)  Indices=1  OutputSizes=1
  Selector1 : Selector  InputPortWidth=3  IndexOptions=Index vector (dialog)  Indices=2  OutputSizes=1
  Selector2 : Selector  InputPortWidth=3  IndexOptions=Index vector (dialog)  Indices=3  OutputSizes=1
  V0/V1 max3 : Constant  Value=Max_I1
  V1 max : Constant  Value=Max_I2_I1
  V1 max2 : Constant  Value=Max_Iinst
  MaxIinst : Outport
  MaxI1 : Outport  Port=2
  MaxI2I1 : Outport  Port=3
  wires:
  abc/1 -> Current Measurement/1(abc), Selector/1, Selector1/1, Selector2/1
  Current Measurement/1(I1) -> Relational Operator6/1
  V0/V1 max3/1 -> Relational Operator6/2
  V1 max/1 -> Relational Operator8/2
  Current Measurement/2(I2/I1) -> Relational Operator8/1
  Relational Operator6/1 -> On Delay/1
  Relational Operator8/1 -> On Delay1/1
  On Delay/1 -> MaxI1/1
  On Delay1/1 -> MaxI2I1/1
  Relational Operator10/1 -> MaxIinst/1
  V1 max2/1 -> Relational Operator10/2
  Selector/1 -> Mux/1
  Selector2/1 -> Mux/3
  Selector1/1 -> Mux/2
  Mux/1 -> Complex to Magnitude-Angle1/1
  Complex to Magnitude-Angle1/1 -> MinMax/1
  MinMax/1 -> Relational Operator10/1

== system power_wind_dfig/Wind Turbine Protection/Protection System/AC Voltage Protection ==
  abc : Inport  PortDimensions=3
  On Delay : powerlib_meascontrol/Logic/On Delay  DelayType=On delay  delay=Delay_V1  ic=0  Ts=0
  On Delay1 : powerlib_meascontrol/Logic/On Delay  DelayType=On delay  delay=Delay_V2_V1  ic=0  Ts=0
  On Delay2 : powerlib_meascontrol/Logic/On Delay  DelayType=On delay  delay=Delay_V1  ic=0  Ts=0
  On Delay3 : powerlib_meascontrol/Logic/On Delay  DelayType=On delay  delay=Delay_V2_V1  ic=0  Ts=0
  Relational Operator6 : RelationalOperator  Operator=>
  Relational Operator7 : RelationalOperator  Operator=<
  Relational Operator8 : RelationalOperator  Operator=>
  Relational Operator9 : RelationalOperator  Operator=>
  V0/V1 max3 : Constant  Value=Max_V1
  V0/V1 max4 : Constant  Value=Min_V1
  V1 max : Constant  Value=Max_V2_V1
  V1 max1 : Constant  Value=Max_V0_V1
  Voltage Measurement : Subsystem
  MinV1 : Outport
  MaxV1 : Outport  Port=2
  MaxV2V1 : Outport  Port=3
  MaxV0V1 : Outport  Port=4
  wires:
  On Delay3/1 -> MaxV0V1/1
  On Delay1/1 -> MaxV2V1/1
  On Delay/1 -> MinV1/1
  On Delay2/1 -> MaxV1/1
  Relational Operator9/1 -> On Delay3/1
  Relational Operator8/1 -> On Delay1/1
  Relational Operator7/1 -> On Delay/1
  Relational Operator6/1 -> On Delay2/1
  Voltage Measurement/3(V0/V1) -> Relational Operator9/1
  V1 max1/1 -> Relational Operator9/2
  Voltage Measurement/2(V2/V1) -> Relational Operator8/1
  V1 max/1 -> Relational Operator8/2
  V0/V1 max4/1 -> Relational Operator7/2
  V0/V1 max3/1 -> Relational Operator6/2
  Voltage Measurement/1(V1) -> Relational Operator7/1, Relational Operator6/1
  abc/1 -> Voltage Measurement/1(abc)

== system power_wind_dfig/Wind Turbine Protection/Protection System/DC Voltage Protection ==
  Vdc : Inport
  On Delay : powerlib_meascontrol/Logic/On Delay  DelayType=On delay  delay=Delay_Vdc  ic=0  Ts=0
  Relational Operator1 : RelationalOperator  Operator=>
  V1 max3 : Constant  Value=Max_Vdc
  MaxVdc : Outport
  wires:
  Vdc/1 -> Relational Operator1/1
  V1 max3/1 -> Relational Operator1/2
  Relational Operator1/1 -> On Delay/1
  On Delay/1 -> MaxVdc/1

== system power_wind_dfig/Wind Turbine Protection/Protection System/Decoding ==
  Code : Inport
  Constant : Constant  Value=pow2(0:-1:-9)
  Constant6 : Constant  Value=2
  Math Function : Math  Operator=rem  SaturateOnIntegerOverflow=on
  Product : Product  SaturateOnIntegerOverflow=on  InputSameDT=on  OutDataTypeStr=Inherit: Same as first input
  Rounding Function : Rounding
  Out : Outport
  wires:
  Constant/1 -> Product/2
  Code/1 -> Product/1
  Product/1 -> Rounding Function/1
  Constant6/1 -> Math Function/2
  Rounding Function/1 -> Math Function/1
  Math Function/1 -> Out/1

== system power_wind_dfig/Wind Turbine Protection/Protection System/Encoding ==
  In1 : Inport
  In2 : Inport  Port=2
  In3 : Inport  Port=3
  In4 : Inport  Port=4
  In5 : Inport  Port=5
  In6 : Inport  Port=6
  In7 : Inport  Port=7
  In8 : Inport  Port=8
  In9 : Inport  Port=9
  In10 : Inport  Port=10
  Constant12 : Constant  Value=pow2(0:1:9)
  Data Type Conversion : DataTypeConversion  SaturateOnIntegerOverflow=on  RndMeth=Zero
  Mux : Mux  Inputs=10
  Product : Product  SaturateOnIntegerOverflow=on  InputSameDT=on  OutDataTypeStr=Inherit: Same as first input
  Sum : Sum  Inputs=1  SaturateOnIntegerOverflow=on  InputSameDT=on  OutDataTypeStr=Inherit: Same as first input
  Code : Outport
  wires:
  Data Type Conversion/1 -> Product/1
  Mux/1 -> Data Type Conversion/1
  In2/1 -> Mux/2
  In3/1 -> Mux/3
  In4/1 -> Mux/4
  In5/1 -> Mux/5
  In6/1 -> Mux/6
  In7/1 -> Mux/7
  In8/1 -> Mux/8
  In9/1 -> Mux/9
  In10/1 -> Mux/10
  In1/1 -> Mux/1
  Product/1 -> Sum/1
  Constant12/1 -> Product/2
  Sum/1 -> Code/1

== system power_wind_dfig/Wind Turbine Protection/Protection System/Sample & Hold ==
  note: Silvano Casoria
      | Power System Simulation Laboratory
      | IREQ, Hydro-Quebc
  note: Sample and Hold
  In : Inport
  S : Inport  Port=2
  IC=ic : Memory  X0=ic  InheritSampleTime=on
  Switch : Switch  Threshold=0.5  SaturateOnIntegerOverflow=on  InputSameDT=on
  "   " : Outport  InitialOutput=0
  wires:
  S/1 -> Switch/2
  In/1 -> Switch/1
  IC=ic/1 -> Switch/3
  Switch/1 -> IC=ic/1, "   "/1

== system power_wind_dfig/Wind Turbine Protection/Protection System/Sample & Hold1 ==
  note: Silvano Casoria
      | Power System Simulation Laboratory
      | IREQ, Hydro-Quebc
  note: Sample and Hold
  In : Inport
  S : Inport  Port=2
  IC=ic : Memory  X0=ic  InheritSampleTime=on
  Switch : Switch  Threshold=0.5  SaturateOnIntegerOverflow=on  InputSameDT=on
  "   " : Outport  InitialOutput=0
  wires:
  S/1 -> Switch/2
  In/1 -> Switch/1
  IC=ic/1 -> Switch/3
  Switch/1 -> IC=ic/1, "   "/1

== system power_wind_dfig/Wind Turbine Protection/Protection System/Under//Over Speed Protection ==
  Speed : Inport  PortDimensions=1
  On Delay : powerlib_meascontrol/Logic/On Delay  DelayType=On delay  delay=Delay_Speed  ic=0  Ts=0
  On Delay1 : powerlib_meascontrol/Logic/On Delay  DelayType=On delay  delay=Delay_Speed  ic=0  Ts=0
  Relational Operator1 : RelationalOperator  Operator=>
  Relational Operator3 : RelationalOperator  Operator=<
  V1 max1 : Constant  Value=Min_Speed
  V1 max3 : Constant  Value=Max_Speed
  MinSpeed : Outport
  MaxSpeed : Outport  Port=2
  wires:
  Relational Operator3/1 -> On Delay/1
  Relational Operator1/1 -> On Delay1/1
  V1 max1/1 -> Relational Operator3/2
  V1 max3/1 -> Relational Operator1/2
  Speed/1 -> Relational Operator3/1, Relational Operator1/1
  On Delay/1 -> MinSpeed/1
  On Delay1/1 -> MaxSpeed/1

== system power_wind_dfig/Measurements/Wind turbine Data acquisition/magnitude positive seq. /Fourier1 ==
  signal : Inport
  Constant : Constant  Value=0
  Fcn : Fcn  Expr=u^2
  Fcn1 : Fcn  Expr=u^2
  Fcn2 : Fcn  Expr=sqrt(u)
  Fcn3 : Fcn  Expr=180/pi*atan2(u[2],u[1])
  Gain1 : Gain  Gain=k*f1  SaturateOnIntegerOverflow=on  OutDataTypeStr=Inherit: Same as input  ParamDataTypeStr=Inherit: Same as input
  Integ2 : Integrator  InitialConditionSource=external
  Mux : Mux  Inputs=2
  Product : Product  SaturateOnIntegerOverflow=on  InputSameDT=on  OutDataTypeStr=Inherit: Same as first input
  Product1 : Product  SaturateOnIntegerOverflow=on  InputSameDT=on  OutDataTypeStr=Inherit: Same as first input
  Sum : Sum  SaturateOnIntegerOverflow=on  InputSameDT=on  OutDataTypeStr=Inherit: Same as first input
  Sum1 : Sum  Inputs=+-  SaturateOnIntegerOverflow=on  InputSameDT=on  OutDataTypeStr=Inherit: Same as first input
  Sum2 : Sum  Inputs=+-  SaturateOnIntegerOverflow=on  InputSameDT=on  OutDataTypeStr=Inherit: Same as first input
  T : TransportDelay  DelayTime=1/f1  BufferSize=2048
  T1 : TransportDelay  DelayTime=1/f1  BufferSize=2048
  cos(nwt) : Sin  Frequency=2*pi*n*f1  Phase=pi/2  SampleTime=0
  integ1 : Integrator  InitialConditionSource=external
  sin(nwt) : Sin  Frequency=2*pi*n*f1  SampleTime=0
  magnitude : Outport  InitialOutput=0
  angle : Outport  Port=2  InitialOutput=0
  wires:
  Constant/1 -> integ1/2, Integ2/2
  Sum/1 -> Fcn2/1
  Fcn/1 -> Sum/1
  Fcn1/1 -> Sum/2
  Mux/1 -> Fcn3/1
  Fcn3/1 -> angle/1
  sin(nwt)/1 -> Product/1
  cos(nwt)/1 -> Product1/2
  Product/1 -> integ1/1
  Product1/1 -> Integ2/1
  T/1 -> Sum1/2
  T1/1 -> Sum2/2
  integ1/1 -> Sum1/1, T/1
  Integ2/1 -> T1/1, Sum2/1
  Sum2/1 -> Fcn1/1, Mux/2
  Sum1/1 -> Fcn/1, Mux/1
  signal/1 -> Gain1/1
  Gain1/1 -> Product/2, Product1/1
  Fcn2/1 -> magnitude/1
